simulink model "Example_1_3"  (R2022b)
settings: Solver=VariableStepAuto  StartTime=0.0  StopTime=150  RelTol=1e-3
settings Model: Creator=USER  LastModifiedBy=USER
settings DataIOCC: Refine=4

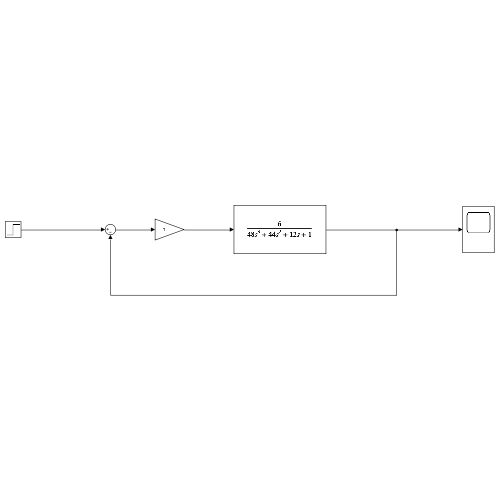
[thumbnail: Simulink's stored preview of the top-level diagram]
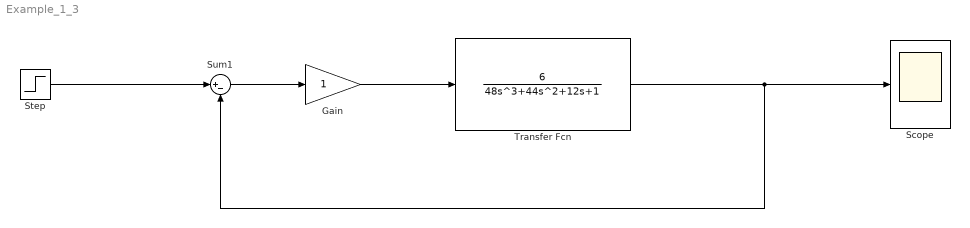
== system Example_1_3 ==
  Gain : Gain
  Scope : Scope
  Step : Step  SampleTime=0
  Sum1 : Sum  Inputs=|+-
  Transfer Fcn : TransferFcn  Numerator=[6]  Denominator=[48 44 12 1]
  wires:
  Transfer Fcn/1 -> Sum1/2, Scope/1
  Gain/1 -> Transfer Fcn/1
  Sum1/1 -> Gain/1
  Step/1 -> Sum1/1
